simulink model "real_plant_v2_22a"  (R2022a)
settings: Solver=FixedStepAuto  StartTime=0.0  StopTime=inf  FixedStep=0.001  RelTol=1e-3  EnableMultiTasking=on
values from neighbouring files (symbols this model uses):
  A = double(A)    [main.m]
  B = double(B)    [main.m]
  C = [1, 0, 0, 0, 0, 0;     0, 1, 0, 0, 0, 0;     0, 0, 1, 0, 0, 0]    [main.m]
  H = place(A', C', P_beo)'    [main.m]
  pos1 = deg2rad([alpha1, beta1; alpha2, beta2; alpha3, beta3])    [main.m]
  pos2 = deg2rad([alpha1, beta1; alpha2, beta2; alpha3, beta3])    [main.m]
  pos3 = deg2rad([alpha1, beta1; alpha2, beta2; alpha3, beta3])    [main.m]
  u_Bs = double(u_s.u_B(1))    [main.m]
  u_Fs = double(u_s.u_F(1))    [main.m]
  x_s = [0, deg2rad(-22), 0, 0, 0, 0]    [main.m]
undefined symbols (not defined in the file or in its folder): HIL, K
libraries: quarc_library x3
settings Model: SimulationMode=external  ExtModeTrigDuration=10000  Creator=student  LastModifiedBy=student
settings SolverCC: AlgebraicLoopSolver=TrustRegion  PositivePriorityOrder=on
settings DataIOCC: ReturnWorkspaceOutputs=off
settings DebuggingCC: UnconnectedInputMsg=warning  UnconnectedOutputMsg=warning  UnconnectedLineMsg=warning  SFMachineParentedDataDiag=warning  ArithmeticOperatorsInVariantConditions=warning
settings SFSimCC: SimUseLocalCustomCode=off  CustomCodeUndefinedFunction=UseInterfaceOnly
settings RTWCC: Description=QUARC Win64 Target Using Toolchain  SystemTargetFile=quarc_win64.tlc  TemplateMakefile=quarc_default_tmf  RTWUseLocalCustomCode=off  Toolchain=QUARC win64 | nmake (64-bit Windows)  BuildConfiguration=Faster Runs
settings CodeAppCC: StateflowObjectComments=on
settings STFCustomTargetCC: TargetLangStandard=C99 (ISO)  ConcurrentExecutionCompliant=on  UseToolchainInfoCompliant=on  SystemTargetFile=quarc_win64.tlc
settings GRTTargetCC: ParMdlRefBuildCompliant=off  CompOptLevelCompliant=off  CombineOutputUpdateFcns=off  MatFileLogging=off  CPPClassGenCompliant=off  GRTInterface=on  ExtMode=on  ExtModeMexFile=quarc_comm
settings ConfigComp: CovMetricSettings=dswe

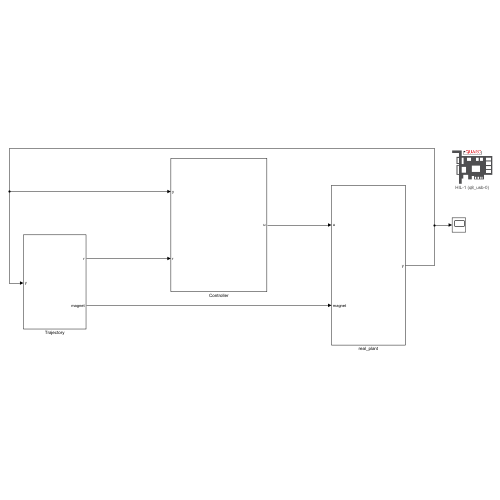
[thumbnail: Simulink's stored preview of the top-level diagram]
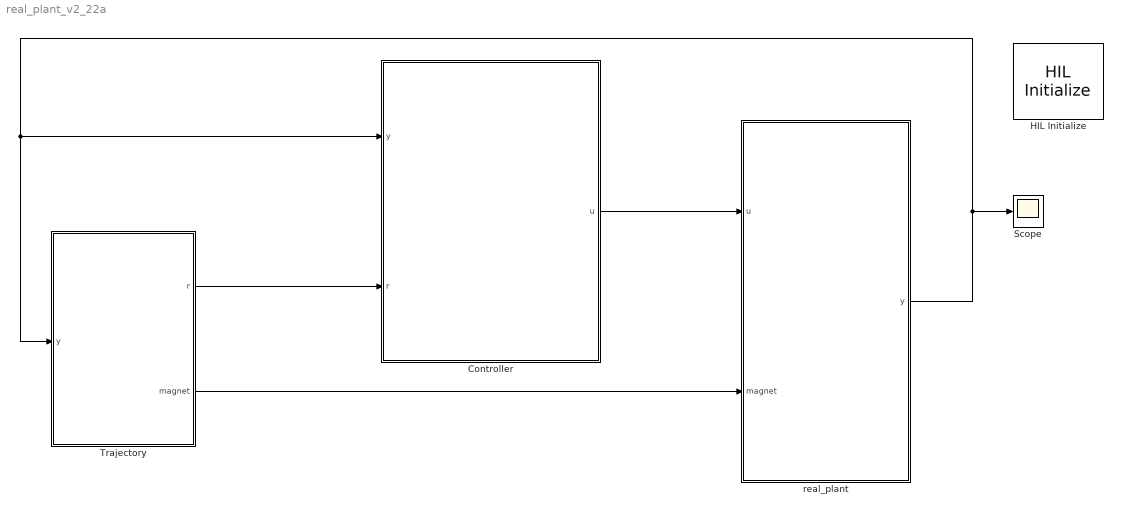
== system real_plant_v2_22a ==
  Controller : Subsystem
  HIL Initialize : quarc_library/Data Acquisition/Generic/Configuration/HIL Initialize  object_name=HIL-1  board_type=q8_usb  board_number=0  board_options=update_rate=normal;decimation=1  exclusive=off  active=on  hardware_clocks=[0:2]  clock_modes=[]  initial_clock_frequencies=[]  set_clock_params_at_start=off  set_clock_params_at_switch_in=off  set_clock_frequencies_at_start=off  set_clock_frequencies_at_switch_in=off  analog_input_channels=[0:7]  analog_input_configurations=[]  analog_input_maximums=10  analog_input_minimums=-10  set_analog_input_params_at_start=on  set_analog_input_params_at_switch_in=off  analog_output_channels=[0:7]  analog_output_maximums=10  analog_output_minimums=-10  initial_analog_outputs=[0]  final_analog_outputs=[0]  watchdog_analog_outputs=0  set_analog_output_params_at_start=on  set_analog_output_params_at_switch_in=off  set_analog_outputs_at_start=on  set_analog_outputs_at_switch_in=off  set_analog_outputs_at_terminate=on  set_analog_outputs_at_switch_out=off  set_analog_outputs_on_watchdog=off  digital_input_channels=[]  digital_output_channels=[]  digital_output_configuration=[]  initial_digital_outputs=[1]  final_digital_outputs=[1]  watchdog_digital_outputs=[1]  set_digital_output_params_at_start=off  set_digital_output_params_at_switch_in=off  set_digital_outputs_at_start=on  set_digital_outputs_at_switch_in=off  set_digital_outputs_at_terminate=on  set_digital_outputs_at_switch_out=off  set_digital_outputs_on_watchdog=off  encoder_channels=[0:7]  quadrature=[4]  encoder_filter_frequency=[]  initial_encoder_counts=[0]  set_encoder_params_at_start=on  set_encoder_params_at_switch_in=off  set_encoder_counts_at_start=on  set_encoder_counts_at_switch_in=off  pwm_channels=[0:7]  pwm_modes=0  pwm_frequency=99.532799999999995e6/4095  pwm_configuration=[0]  pwm_alignment=[0]  pwm_polarity=[1]  pwm_leading_deadband=[0]  pwm_trailing_deadband=[0]  initial_pwm_outputs=[0]  final_pwm_outputs=[0]  watchdog_pwm_outputs=[0]  set_pwm_params_at_start=on  set_pwm_params_at_switch_in=off  set_pwm_outputs_at_start=on  set_pwm_outputs_at_switch_in=off  set_pwm_outputs_at_terminate=on  set_pwm_outputs_at_switch_out=off  set_pwm_outputs_on_watchdog=off  other_output_channels=[]  initial_other_outputs=[]  final_other_outputs=[]  watchdog_other_outputs=[]  set_other_outputs_at_start=off  set_other_outputs_at_switch_in=off  set_other_outputs_at_terminate=off  set_other_outputs_at_switch_out=off  set_other_outputs_on_watchdog=off
  Scope : Scope
  Trajectory : Subsystem
  real_plant : Subsystem
  wires:
  real_plant/1(y) -> Controller/1(y), Trajectory/1(y), Scope/1
  Controller/1(u) -> real_plant/1(u)
  Trajectory/1(r) -> Controller/2(r)
  Trajectory/2(magnet) -> real_plant/2(magnet)

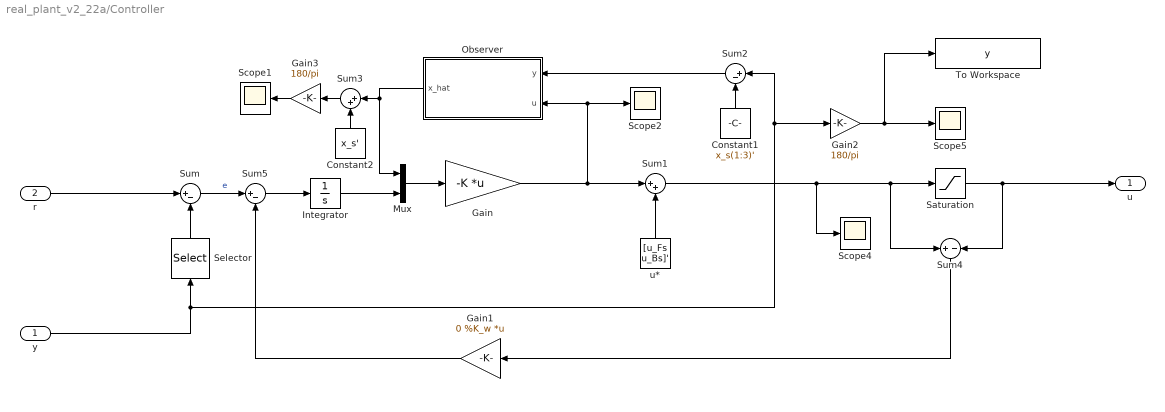
== system real_plant_v2_22a/Controller ==
  y : Inport
  r : Inport  Port=2
  Constant1 : Constant  Value=x_s(1:3)'
  Constant2 : Constant  Value=x_s'
  Gain : Gain  Gain=-K  Multiplication=Matrix(K*u) (u vector)
  Gain1 : Gain  Gain=0 %K_w  Multiplication=Matrix(K*u)
  Gain2 : Gain  Gain=180/pi
  Gain3 : Gain  Gain=180/pi
  Integrator : Integrator  InitialCondition=[0; -0.1675]
  Mux : Mux  Inputs=2
  Observer : Subsystem
  Saturation : Saturate  UpperLimit=[4 4]  LowerLimit=[-4 -4]
  Scope{1..2,4..5} (4 alike) : Scope
  Selector : Selector  InputPortWidth=3  IndexOptions=Index vector (dialog)  Indices=[1 2]  OutputSizes=1
  Sum : Sum  Inputs=|+-
  Sum1 : Sum  Inputs=|++
  Sum2 : Sum  Inputs=|+-
  Sum3 : Sum  Inputs=|++
  Sum4 : Sum  Inputs=+|-
  Sum5 : Sum  Inputs=|+-
  To Workspace : ToWorkspace  VariableName=y  SampleTime=-1
  u* : Constant  Value=[u_Fs u_Bs]'
  u : Outport
  wires:
  Integrator/1 -> Mux/2
  Constant2/1 -> Sum3/2
  Sum1/1 -> Sum4/1, Saturation/1, Scope4/1
  Mux/1 -> Gain/1
  Sum4/1 -> Gain1/1
  Gain3/1 -> Scope1/1
  Selector/1 -> Sum/2
  Gain/1 -> Scope2/1, Observer/2(u), Sum1/1
  Sum2/1 -> Observer/1(y)
  Observer/1(x_hat) -> Sum3/1, Mux/1
  r/1 -> Sum/1
  Sum/1 -> Sum5/1  "e"
  Sum3/1 -> Gain3/1
  Gain2/1 -> Scope5/1, To Workspace/1
  Constant1/1 -> Sum2/2
  Saturation/1 -> Sum4/2, u/1
  u*/1 -> Sum1/2
  Sum5/1 -> Integrator/1
  Gain1/1 -> Sum5/2
  y/1 -> Selector/1, Gain2/1, Sum2/1

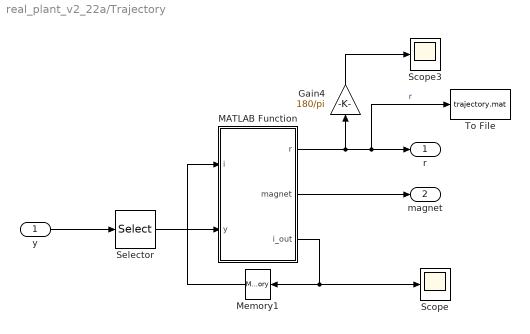
== system real_plant_v2_22a/Trajectory ==
  y : Inport
  Gain4 : Gain  Gain=180/pi
  MATLAB Function : MATLAB Function  TreatAsAtomicUnit=on
  Memory1 : Memory  InitialCondition=1
  Scope : Scope
  Scope3 : Scope
  Selector : Selector  InputPortWidth=3  IndexOptions=Index vector (dialog)  Indices=[1 2]  OutputSizes=1
  To File : ToFile  Filename=trajectory.mat  MatrixName=r
  r : Outport
  magnet : Outport  Port=2
  wires:
  Memory1/1 -> MATLAB Function/1(i)
  MATLAB Function/3(i_out) -> Memory1/1, Scope/1
  Gain4/1 -> Scope3/1
  MATLAB Function/1(r) -> To File/1, r/1, Gain4/1  "r"
  y/1 -> Selector/1
  Selector/1 -> MATLAB Function/2(y)
  MATLAB Function/2(magnet) -> magnet/1

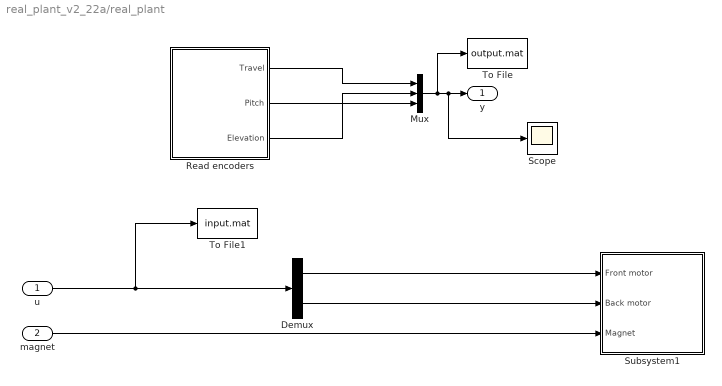
== system real_plant_v2_22a/real_plant ==
  u : Inport
  magnet : Inport  Port=2
  Demux : Demux  Outputs=2
  Mux : Mux  Inputs=3
  Read encoders : Subsystem
  Scope : Scope
  Subsystem1 : Subsystem
  To File : ToFile  Filename=output.mat  MatrixName=y
  To File1 : ToFile  Filename=input.mat  MatrixName=u
  y : Outport
  wires:
  Read encoders/1(Travel) -> Mux/1
  u/1 -> To File1/1, Demux/1
  magnet/1 -> Subsystem1/3(Magnet)
  Mux/1 -> To File/1, Scope/1, y/1
  Read encoders/3(Elevation) -> Mux/2
  Read encoders/2(Pitch) -> Mux/3
  Demux/1 -> Subsystem1/1(Front motor)
  Demux/2 -> Subsystem1/2(Back motor)

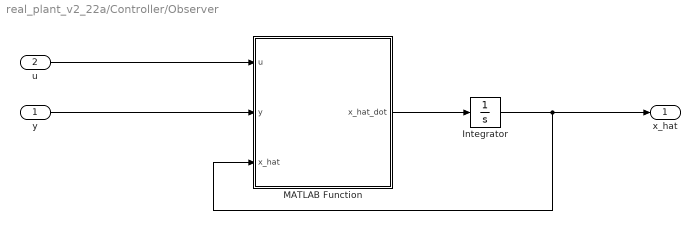
== system real_plant_v2_22a/Controller/Observer ==
  y : Inport
  u : Inport  Port=2
  Integrator : Integrator  InitialCondition=deg2rad([0; -5; 0; 0; 0; 0])
  MATLAB Function : MATLAB Function  TreatAsAtomicUnit=on
  x_hat : Outport
  wires:
  MATLAB Function/1(x_hat_dot) -> Integrator/1
  Integrator/1 -> x_hat/1, MATLAB Function/3(x_hat)
  u/1 -> MATLAB Function/1(u)
  y/1 -> MATLAB Function/2(y)

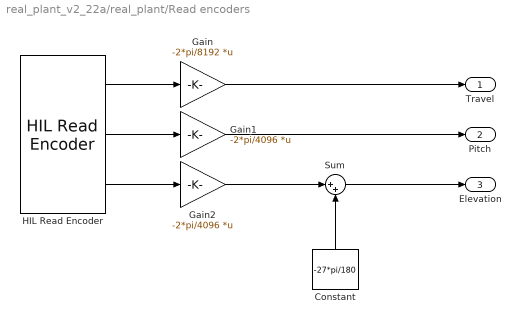
== system real_plant_v2_22a/real_plant/Read encoders ==
  Constant : Constant  Value=-27*pi/180
  Gain : Gain  Gain=-2*pi/8192  Multiplication=Matrix(K*u)
  Gain1 : Gain  Gain=-2*pi/4096  Multiplication=Matrix(K*u)
  Gain2 : Gain  Gain=-2*pi/4096  Multiplication=Matrix(K*u)
  HIL Read Encoder : quarc_library/Data Acquisition/Generic/Immediate I//O/HIL Read Encoder  object_name=HIL-1  channels=[0:2]  sample_time=qc_get_step_size  active=on  vector_output=off  data_type_mode=Inherit via back propagation  data_type=double
  Sum : Sum  Inputs=|++
  Travel : Outport
  Pitch : Outport  Port=2
  Elevation : Outport  Port=3
  wires:
  HIL Read Encoder/1 -> Gain/1
  HIL Read Encoder/2 -> Gain1/1
  HIL Read Encoder/3 -> Gain2/1
  Gain/1 -> Travel/1
  Gain1/1 -> Pitch/1
  Sum/1 -> Elevation/1
  Gain2/1 -> Sum/1
  Constant/1 -> Sum/2

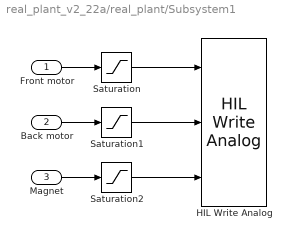
== system real_plant_v2_22a/real_plant/Subsystem1 ==
  Front motor : Inport
  Back motor : Inport  Port=2
  Magnet : Inport  Port=3
  HIL Write Analog : quarc_library/Data Acquisition/Generic/Immediate I//O/HIL Write Analog  object_name=HIL-1  channels=[0:2]  sample_time=-1  active=off  vector_input=off
  Saturation : Saturate  UpperLimit=4  LowerLimit=-4
  Saturation1 : Saturate  UpperLimit=4  LowerLimit=-4
  Saturation2 : Saturate  UpperLimit=1  LowerLimit=0
  wires:
  Magnet/1 -> Saturation2/1
  Front motor/1 -> Saturation/1
  Back motor/1 -> Saturation1/1
  Saturation1/1 -> HIL Write Analog/2
  Saturation/1 -> HIL Write Analog/1
  Saturation2/1 -> HIL Write Analog/3

== matlab function real_plant_v2_22a/Controller/Observer/MATLAB Function ==
  data: u input; x_hat_dot output; y input; x_hat input; A parameter; B parameter; C parameter; H parameter
function x_hat_dot = fcn(u, y, x_hat, A, B, C, H)
    x_hat_dot = A*x_hat + B*u + H*(y-C*x_hat);
end

== matlab function real_plant_v2_22a/Trajectory/MATLAB Function ==
  data: i input; r output; magnet output; pos1 parameter; pos2 parameter; i_out output; y input; pos3 parameter
function [r, magnet, i_out] = fcn(i, pos1, pos2, y, pos3)
    epsilon1 = deg2rad(2); 
    epsilon2 = deg2rad(2.5); 
    if i < size(pos1, 1)
        r = pos1(i,:)';
        i_out = i+1;
        magnet = 0;
    elseif i == size(pos1,1)
        if abs(y(1)-pos1(end,1)) > epsilon1 || abs(y(2)-pos1(end,2)) > epsilon2
            %rad2deg(norm(y-pos1(end,:)'))
            r = pos1(end,:)';
            %disp('let''s catch the ball!');
            i_out = i;
            magnet = 1;
        else
            i_out = i+1;
            r = pos1(end,:)';
            magnet = 1;
        end
    elseif i< size(pos1, 1)+ size(pos2,1)
        r = pos2(i-size(pos1, 1),:)';
        i_out = i+1;
        magnet = 1;
    elseif i == size(pos1, 1) + size(pos2,1)
       if abs(y(1)-pos2(end,1)) > epsilon1 || abs(y(2)-pos2(end,2)) > epsilon2
            %rad2deg(norm(y-pos2(end,:)'))
            r = pos2(end,:)';
            %disp('let''s place the ball!');
            i_out = i;
            magnet = 1;
       else
            magnet = 0;
            i_out = i+1;
            r = pos2(end,:)';
       end
    elseif i < size(pos1, 1) + size(pos2,1) + size(pos3,1)
        r = pos3(i-size(pos1, 1)-size(pos2,1),:)';
        i_out = i+1;
        magnet = 0;
    else 
        r = pos3(end,:)';
        i_out = i;
        magnet = 0;
    end
